simulink model "Casc_Filter_x4"  (Simulink 6.6)
settings: Solver=ode45  StartTime=0.0  StopTime=4100/sampling_freq  RelTol=1e-3
values from neighbouring files (symbols this model uses):
  filter_clk = sampling_freq*clk_mult    (= 144000000)    [Casecade_Taps.m]
  h_g = round(h_g*2^17)/2^17    [Casecade_Taps.m]
  h_k = round(h_k*2^17)/2^17    [Casecade_Taps.m]
  sampling_freq = 48e6    (= 48000000)    [Casecade_Taps.m]
undefined symbols (not defined in the file or in its folder): A, B, Fs, get, PCIN
libraries: xbsIndex_r4 x839, dspsnks4 x5, dspsrcs4 x1, simulink x1
(part 1 of 8)
settings Model: Creator=tbrimeye  LastModifiedBy=tbrimeye
settings DebuggingCC: SignalResolutionControl=TryResolveAllWithWarning  MultiTaskDSMMsg=warning  MultiTaskCondExecSysMsg=none
settings RTWCC: IncludeERTFirstTime=on

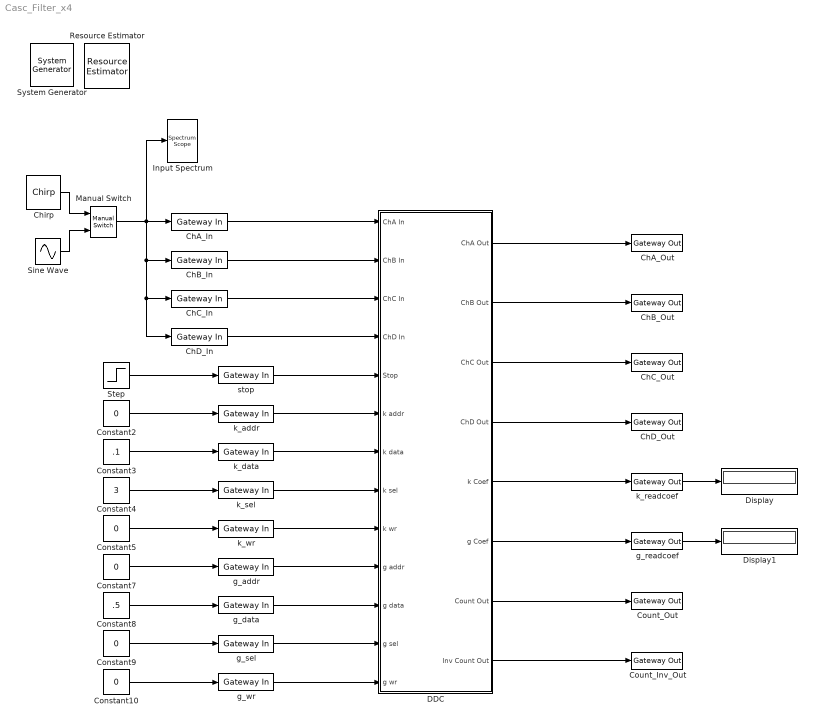
== system Casc_Filter_x4 ==
  " System Generator" : xbsIndex_r4/ System Generator  Tag=genX  SystemSampleTime=-1  xilinxfamily=virtex4  part=xc4vsx35  speed=-11  package=ff668  synthesis_tool=XST  directory=C:/Work_Projects/Xilinx/SysGen_Outputs/DDC_Filters/Casc_Filter_x4_Temp  testbench=off  simulink_period=1/filter_clk  sysclk_period=(1/filter_clk)*1e9  incr_netlist=off  trim_vbits=Everywhere in SubSystem  dbl_ovrd=According to Block Masks  core_generation=According to Block Masks  run_coregen=off  deprecated_control=off  eval_field=0  block_type=sysgen
      settings: block_version=8.2
  ChA_In : xbsIndex_r4/Gateway In  arith_type="Signed  (2's comp)"  n_bits=14  bin_pt=13  quantization="Round  (unbiased: +/- Inf)"  overflow=Saturate  period=1/sampling_freq  dbl_ovrd=off  timing_constraint=None  locs_specified=off  LOCs={}  block_type=gatewayin
      settings: infoedit="Gateway in block.  Converts inputs of type Simulink integer, double and fixed point to  Xilinx fixed point type.<P><P>Hardware notes:  In hardware these blocks become top level input ports."  xl_area=[0 0 0 0 14 0 0]  block_version=8.2
  ChA_Out : xbsIndex_r4/Gateway Out  hdl_port=on  timing_constraint=None  locs_specified=off  LOCs={}  block_type=gatewayout
      settings: infoedit="Gateway out block.  Converts Xilinx fixed point inputs into ouputs of type Simulink integer, double, or fixed point.<P><P>Hardware notes:  In hardware these blocks become top level output ports or are discarded, depending on how they are configured."  xl_area=[0 0 0 0 16 0 0]  block_version=8.2
  ChB_In : xbsIndex_r4/Gateway In  arith_type="Signed  (2's comp)"  n_bits=14  bin_pt=13  quantization="Round  (unbiased: +/- Inf)"  overflow=Saturate  period=1/sampling_freq  dbl_ovrd=off  timing_constraint=None  locs_specified=off  LOCs={}  block_type=gatewayin
      settings: infoedit="Gateway in block.  Converts inputs of type Simulink integer, double and fixed point to  Xilinx fixed point type.<P><P>Hardware notes:  In hardware these blocks become top level input ports."  xl_area=[0 0 0 0 14 0 0]  block_version=8.2
  ChB_Out : xbsIndex_r4/Gateway Out  hdl_port=on  timing_constraint=None  locs_specified=off  LOCs={}  block_type=gatewayout
      settings: infoedit="Gateway out block.  Converts Xilinx fixed point inputs into ouputs of type Simulink integer, double, or fixed point.<P><P>Hardware notes:  In hardware these blocks become top level output ports or are discarded, depending on how they are configured."  xl_area=[0 0 0 0 16 0 0]  block_version=8.2
  ChC_In : xbsIndex_r4/Gateway In  arith_type="Signed  (2's comp)"  n_bits=14  bin_pt=13  quantization="Round  (unbiased: +/- Inf)"  overflow=Saturate  period=1/sampling_freq  dbl_ovrd=off  timing_constraint=None  locs_specified=off  LOCs={}  block_type=gatewayin
      settings: infoedit="Gateway in block.  Converts inputs of type Simulink integer, double and fixed point to  Xilinx fixed point type.<P><P>Hardware notes:  In hardware these blocks become top level input ports."  xl_area=[0 0 0 0 14 0 0]  block_version=8.2
  ChC_Out : xbsIndex_r4/Gateway Out  hdl_port=on  timing_constraint=None  locs_specified=off  LOCs={}  block_type=gatewayout
      settings: infoedit="Gateway out block.  Converts Xilinx fixed point inputs into ouputs of type Simulink integer, double, or fixed point.<P><P>Hardware notes:  In hardware these blocks become top level output ports or are discarded, depending on how they are configured."  xl_area=[0 0 0 0 16 0 0]  block_version=8.2
  ChD_In : xbsIndex_r4/Gateway In  arith_type="Signed  (2's comp)"  n_bits=14  bin_pt=13  quantization="Round  (unbiased: +/- Inf)"  overflow=Saturate  period=1/sampling_freq  dbl_ovrd=off  timing_constraint=None  locs_specified=off  LOCs={}  block_type=gatewayin
      settings: infoedit="Gateway in block.  Converts inputs of type Simulink integer, double and fixed point to  Xilinx fixed point type.<P><P>Hardware notes:  In hardware these blocks become top level input ports."  xl_area=[0 0 0 0 14 0 0]  block_version=8.2
  ChD_Out : xbsIndex_r4/Gateway Out  hdl_port=on  timing_constraint=None  locs_specified=off  LOCs={}  block_type=gatewayout
      settings: infoedit="Gateway out block.  Converts Xilinx fixed point inputs into ouputs of type Simulink integer, double, or fixed point.<P><P>Hardware notes:  In hardware these blocks become top level output ports or are discarded, depending on how they are configured."  xl_area=[0 0 0 0 16 0 0]  block_version=8.2
  Chirp : dspsrcs4/Chirp  sweep=Linear  mode=Unidirectional  f0=0  f1=sampling_freq_div2  t1=4096/sampling_freq  Tsweep=4096/sampling_freq  phase=pi/4  Ts=1/sampling_freq  spf=1  datatype=Double
  Constant{2,5,7,9..10} (5 alike) : Constant  Value=0
  Constant3 : Constant  Value=.1
  Constant4 : Constant  Value=3
  Constant8 : Constant  Value=.5
  Count_Inv_Out : xbsIndex_r4/Gateway Out  hdl_port=on  timing_constraint=None  locs_specified=off  LOCs={}  block_type=gatewayout
      settings: infoedit="Gateway out block.  Converts Xilinx fixed point inputs into ouputs of type Simulink integer, double, or fixed point.<P><P>Hardware notes:  In hardware these blocks become top level output ports or are discarded, depending on how they are configured."  xl_area=[0 0 0 0 16 0 0]  block_version=8.2
  Count_Out : xbsIndex_r4/Gateway Out  hdl_port=on  timing_constraint=None  locs_specified=off  LOCs={}  block_type=gatewayout
      settings: infoedit="Gateway out block.  Converts Xilinx fixed point inputs into ouputs of type Simulink integer, double, or fixed point.<P><P>Hardware notes:  In hardware these blocks become top level output ports or are discarded, depending on how they are configured."  xl_area=[0 0 0 0 16 0 0]  block_version=8.2
  DDC : Subsystem
  Display : Display
  Display1 : Display
  Input Spectrum : dspsnks4/Spectrum Scope  DialogController=dspdialog.SpectrumScope  DialogControllerArgs=DataTag5  SystemSampleTime=-1  ScopeProperties=on  Domain=Frequency  HorizSpan=1  UseBuffer=on  BufferSize=4096  Overlap=64  inpFftLenInherit=on  FFTlength=4096  numAvg=2  DisplayProperties=off  AxisGrid=on  Memory=off  FrameNumber=on  AxisLegend=off  AxisZoom=off  OpenScopeAtSimStart=on  OpenScopeImmediately=off  FigPos=get(0,'defaultfigureposition')  AxisProperties=off  XUnits=Hertz  XRange=[-Fs/2...Fs/2]  InheritXIncr=on  XIncr=1.0  XLabel=Samples  XLimit=Auto  YUnits=dB  XMax=1  XMin=0  YLabel=Magnitude-squared, dB  LineProperties=off  wintypeSpecScope=Boxcar  RsSpecScope=50  betaSpecScope=5  winsampSpecScope=Periodic
      settings: YMin=-100  YMax=0
  Manual Switch : simulink/Signal Routing/Manual Switch  SystemSampleTime=-1  sw=1  action=0  varsize=off
  Resource Estimator : xbsIndex_r4/Resource Estimator  Tag=resEstTag  Slices=925  FFs=1405  BRAMs=7  LUTs=1104  IOBs=133  EBMs=14  TBUFs=0  xl_use_estimator_area=off  est_options=Post Map  xl_estimator_area=[1915 2342 0 3405 33 4 0]  block_type=resource_estimator
      settings: AttributesFormatString=Resource\nEstimator  block_version=8.2
  Sine Wave : Sin  Amplitude=.99  Frequency=2*pi*61e6  SampleTime=1/48e6
  Step : Step  Time=101/filter_clk  Before=1  After=0  SampleTime=1/filter_clk
  g_addr : xbsIndex_r4/Gateway In  arith_type=Unsigned  n_bits=4  bin_pt=0  quantization="Round  (unbiased: +/- Inf)"  overflow=Saturate  period=1/sampling_freq  dbl_ovrd=off  timing_constraint=None  locs_specified=off  LOCs={}  block_type=gatewayin
      settings: infoedit="Gateway in block.  Converts inputs of type Simulink integer, double and fixed point to  Xilinx fixed point type.<P><P>Hardware notes:  In hardware these blocks become top level input ports."  xl_area=[0 0 0 0 4 0 0]  block_version=VER_STRING_GOES_HERE
  g_data : xbsIndex_r4/Gateway In  arith_type="Signed  (2's comp)"  n_bits=18  bin_pt=17  quantization="Round  (unbiased: +/- Inf)"  overflow=Saturate  period=1/sampling_freq  dbl_ovrd=off  timing_constraint=None  locs_specified=off  LOCs={}  block_type=gatewayin
      settings: infoedit="Gateway in block.  Converts inputs of type Simulink integer, double and fixed point to  Xilinx fixed point type.<P><P>Hardware notes:  In hardware these blocks become top level input ports."  xl_area=[0 0 0 0 18 0 0]  block_version=VER_STRING_GOES_HERE
  g_readcoef : xbsIndex_r4/Gateway Out  hdl_port=on  timing_constraint=None  locs_specified=off  LOCs={}  block_type=gatewayout
      settings: infoedit="Gateway out block.  Converts Xilinx fixed point inputs into ouputs of type Simulink integer, double, or fixed point.<P><P>Hardware notes:  In hardware these blocks become top level output ports or are discarded, depending on how they are configured."  xl_area=[0 0 0 0 18 0 0]  block_version=VER_STRING_GOES_HERE
  g_sel : xbsIndex_r4/Gateway In  arith_type=Unsigned  n_bits=2  bin_pt=0  quantization="Round  (unbiased: +/- Inf)"  overflow=Saturate  period=1/sampling_freq  dbl_ovrd=off  timing_constraint=None  locs_specified=off  LOCs={}  block_type=gatewayin
      settings: infoedit="Gateway in block.  Converts inputs of type Simulink integer, double and fixed point to  Xilinx fixed point type.<P><P>Hardware notes:  In hardware these blocks become top level input ports."  xl_area=[0 0 0 0 2 0 0]  block_version=VER_STRING_GOES_HERE
  g_wr : xbsIndex_r4/Gateway In  arith_type=Boolean  n_bits=4  bin_pt=0  quantization="Round  (unbiased: +/- Inf)"  overflow=Saturate  period=1/sampling_freq  dbl_ovrd=off  timing_constraint=None  locs_specified=off  LOCs={}  block_type=gatewayin
      settings: infoedit="Gateway in block.  Converts inputs of type Simulink integer, double and fixed point to  Xilinx fixed point type.<P><P>Hardware notes:  In hardware these blocks become top level input ports."  xl_area=[0 0 0 0 1 0 0]  block_version=VER_STRING_GOES_HERE
  k_addr : xbsIndex_r4/Gateway In  arith_type=Unsigned  n_bits=4  bin_pt=0  quantization="Round  (unbiased: +/- Inf)"  overflow=Saturate  period=1/sampling_freq  dbl_ovrd=off  timing_constraint=None  locs_specified=off  LOCs={}  block_type=gatewayin
      settings: infoedit="Gateway in block.  Converts inputs of type Simulink integer, double and fixed point to  Xilinx fixed point type.<P><P>Hardware notes:  In hardware these blocks become top level input ports."  xl_area=[0 0 0 0 4 0 0]  block_version=VER_STRING_GOES_HERE
  k_data : xbsIndex_r4/Gateway In  arith_type="Signed  (2's comp)"  n_bits=18  bin_pt=17  quantization="Round  (unbiased: +/- Inf)"  overflow=Saturate  period=1/sampling_freq  dbl_ovrd=off  timing_constraint=None  locs_specified=off  LOCs={}  block_type=gatewayin
      settings: infoedit="Gateway in block.  Converts inputs of type Simulink integer, double and fixed point to  Xilinx fixed point type.<P><P>Hardware notes:  In hardware these blocks become top level input ports."  xl_area=[0 0 0 0 18 0 0]  block_version=VER_STRING_GOES_HERE
  k_readcoef : xbsIndex_r4/Gateway Out  hdl_port=on  timing_constraint=None  locs_specified=off  LOCs={}  block_type=gatewayout
      settings: infoedit="Gateway out block.  Converts Xilinx fixed point inputs into ouputs of type Simulink integer, double, or fixed point.<P><P>Hardware notes:  In hardware these blocks become top level output ports or are discarded, depending on how they are configured."  xl_area=[0 0 0 0 18 0 0]  block_version=VER_STRING_GOES_HERE
  k_sel : xbsIndex_r4/Gateway In  arith_type=Unsigned  n_bits=2  bin_pt=0  quantization="Round  (unbiased: +/- Inf)"  overflow=Saturate  period=1/sampling_freq  dbl_ovrd=off  timing_constraint=None  locs_specified=off  LOCs={}  block_type=gatewayin
      settings: infoedit="Gateway in block.  Converts inputs of type Simulink integer, double and fixed point to  Xilinx fixed point type.<P><P>Hardware notes:  In hardware these blocks become top level input ports."  xl_area=[0 0 0 0 2 0 0]  block_version=VER_STRING_GOES_HERE
  k_wr : xbsIndex_r4/Gateway In  arith_type=Boolean  n_bits=4  bin_pt=0  quantization="Round  (unbiased: +/- Inf)"  overflow=Saturate  period=1/sampling_freq  dbl_ovrd=off  timing_constraint=None  locs_specified=off  LOCs={}  block_type=gatewayin
      settings: infoedit="Gateway in block.  Converts inputs of type Simulink integer, double and fixed point to  Xilinx fixed point type.<P><P>Hardware notes:  In hardware these blocks become top level input ports."  xl_area=[0 0 0 0 1 0 0]  block_version=VER_STRING_GOES_HERE
  stop : xbsIndex_r4/Gateway In  arith_type=Unsigned  n_bits=1  bin_pt=0  quantization="Round  (unbiased: +/- Inf)"  overflow=Saturate  period=1/12e6  dbl_ovrd=off  timing_constraint=None  locs_specified=off  LOCs={}  block_type=gatewayin
      settings: infoedit="Gateway in block.  Converts inputs of type Simulink integer, double and fixed point to  Xilinx fixed point type.<P><P>Hardware notes:  In hardware these blocks become top level input ports."  xl_area=[0 0 0 0 1 0 0]  block_version=VER_STRING_GOES_HERE
  wires:
  Chirp/1 -> Manual Switch/1
  Sine Wave/1 -> Manual Switch/2
  ChA_In/1 -> DDC/1(ChA In)
  Manual Switch/1 -> Input Spectrum/1, ChA_In/1, ChB_In/1, ChC_In/1, ChD_In/1
  k_sel/1 -> DDC/8(k sel)
  k_addr/1 -> DDC/6(k addr)
  k_data/1 -> DDC/7(k data)
  k_wr/1 -> DDC/9(k wr)
  DDC/5(k Coef) -> k_readcoef/1
  Constant2/1 -> k_addr/1
  Constant3/1 -> k_data/1
  Constant4/1 -> k_sel/1
  Constant5/1 -> k_wr/1
  k_readcoef/1 -> Display/1
  g_readcoef/1 -> Display1/1
  DDC/6(g Coef) -> g_readcoef/1
  g_addr/1 -> DDC/10(g addr)
  g_data/1 -> DDC/11(g data)
  g_sel/1 -> DDC/12(g sel)
  g_wr/1 -> DDC/13(g wr)
  Constant7/1 -> g_addr/1
  Constant8/1 -> g_data/1
  Constant9/1 -> g_sel/1
  Constant10/1 -> g_wr/1
  DDC/1(ChA Out) -> ChA_Out/1
  stop/1 -> DDC/5(Stop)
  DDC/2(ChB Out) -> ChB_Out/1
  DDC/4(ChD Out) -> ChD_Out/1
  DDC/3(ChC Out) -> ChC_Out/1
  ChB_In/1 -> DDC/2(ChB In)
  ChC_In/1 -> DDC/3(ChC In)
  ChD_In/1 -> DDC/4(ChD In)
  Step/1 -> stop/1
  DDC/7(Count Out) -> Count_Out/1
  DDC/8(Inv Count Out) -> Count_Inv_Out/1

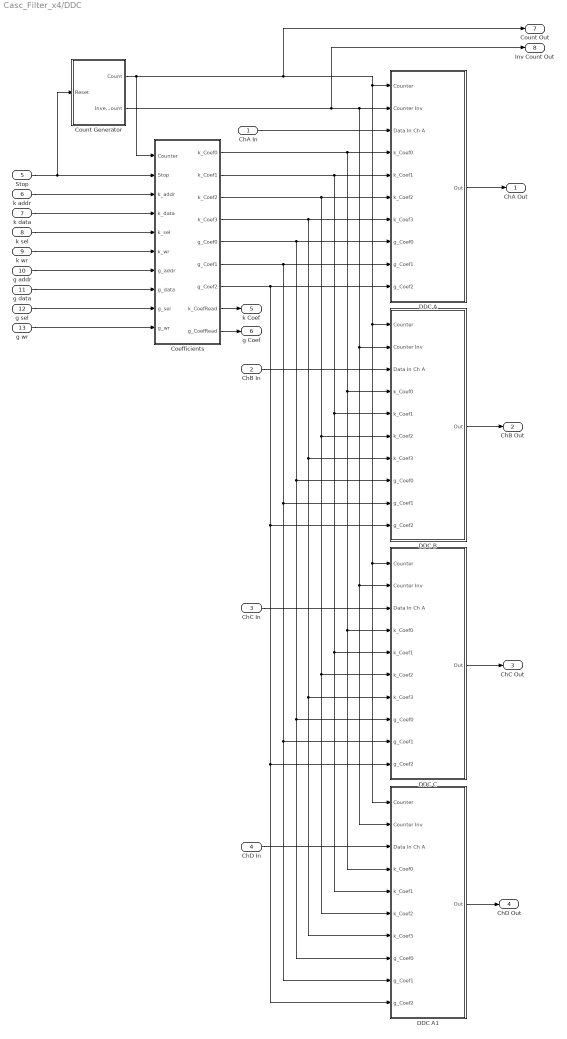
== system Casc_Filter_x4/DDC ==
  ChA In : Inport
  ChB In : Inport  Port=2
  ChC In : Inport  Port=3
  ChD In : Inport  Port=4
  Stop : Inport  Port=5
  k addr : Inport  Port=6
  k data : Inport  Port=7
  k sel : Inport  Port=8
  k wr : Inport  Port=9
  g addr : Inport  Port=10
  g data : Inport  Port=11
  g sel : Inport  Port=12
  g wr : Inport  Port=13
  Coefficients : Subsystem
  Count Generator : Subsystem
  DDC A : Subsystem
  DDC A1 : Subsystem
  DDC B : Subsystem
  DDC C : Subsystem
  ChA Out : Outport
  ChB Out : Outport  Port=2
  ChC Out : Outport  Port=3
  ChD Out : Outport  Port=4
  k Coef : Outport  Port=5
  g Coef : Outport  Port=6
  Count Out : Outport  Port=7
  Inv Count Out : Outport  Port=8
  wires:
  Count Generator/1(Count) -> Coefficients/1(Counter), DDC C/1(Counter), DDC A1/1(Counter), DDC B/1(Counter), DDC A/1(Counter), Count Out/1
  Coefficients/1(k_Coef0) -> DDC C/4(k_Coef0), DDC A1/4(k_Coef0), DDC B/4(k_Coef0), DDC A/4(k_Coef0)
  Coefficients/2(k_Coef1) -> DDC C/5(k_Coef1), DDC A1/5(k_Coef1), DDC B/5(k_Coef1), DDC A/5(k_Coef1)
  Coefficients/3(k_Coef2) -> DDC C/6(k_Coef2), DDC A1/6(k_Coef2), DDC B/6(k_Coef2), DDC A/6(k_Coef2)
  Coefficients/4(k_Coef3) -> DDC C/7(k_Coef3), DDC A1/7(k_Coef3), DDC B/7(k_Coef3), DDC A/7(k_Coef3)
  Count Generator/2(Invert Count) -> DDC C/2(Counter Inv), DDC A1/2(Counter Inv), DDC B/2(Counter Inv), DDC A/2(Counter Inv), Inv Count Out/1
  Coefficients/5(g_Coef0) -> DDC C/8(g_Coef0), DDC A1/8(g_Coef0), DDC B/8(g_Coef0), DDC A/8(g_Coef0)
  Coefficients/6(g_Coef1) -> DDC C/9(g_Coef1), DDC A1/9(g_Coef1), DDC B/9(g_Coef1), DDC A/9(g_Coef1)
  Coefficients/7(g_Coef2) -> DDC C/10(g_Coef2), DDC A1/10(g_Coef2), DDC B/10(g_Coef2), DDC A/10(g_Coef2)
  ChA In/1 -> DDC A/3(Data In Ch A)
  Stop/1 -> Coefficients/2(Stop), Count Generator/1(Reset)
  k addr/1 -> Coefficients/3(k_addr)
  k data/1 -> Coefficients/4(k_data)
  k sel/1 -> Coefficients/5(k_sel)
  k wr/1 -> Coefficients/6(k_wr)
  g addr/1 -> Coefficients/7(g_addr)
  g data/1 -> Coefficients/8(g_data)
  Coefficients/8(k_CoefRead) -> k Coef/1
  g sel/1 -> Coefficients/9(g_sel)
  g wr/1 -> Coefficients/10(g_wr)
  Coefficients/9(g_CoefRead) -> g Coef/1
  DDC A/1(Out) -> ChA Out/1
  DDC B/1(Out) -> ChB Out/1
  DDC C/1(Out) -> ChC Out/1
  DDC A1/1(Out) -> ChD Out/1
  ChB In/1 -> DDC B/3(Data In Ch A)
  ChC In/1 -> DDC C/3(Data In Ch A)
  ChD In/1 -> DDC A1/3(Data In Ch A)

== system Casc_Filter_x4/DDC/Coefficients ==
  Counter : Inport
  Stop : Inport  Port=2
  k_addr : Inport  Port=3
  k_data : Inport  Port=4
  k_sel : Inport  Port=5
  k_wr : Inport  Port=6
  g_addr : Inport  Port=7
  g_data : Inport  Port=8
  g_sel : Inport  Port=9
  g_wr : Inport  Port=10
  Gaus Coef Mem : Subsystem
  Poly Coef Mem : Subsystem
  k_Coef0 : Outport
  k_Coef1 : Outport  Port=2
  k_Coef2 : Outport  Port=3
  k_Coef3 : Outport  Port=4
  g_Coef0 : Outport  Port=5
  g_Coef1 : Outport  Port=6
  g_Coef2 : Outport  Port=7
  k_CoefRead : Outport  Port=8
  g_CoefRead : Outport  Port=9
  wires:
  Stop/1 -> Gaus Coef Mem/1(Stop), Poly Coef Mem/1(Stop)
  Counter/1 -> Poly Coef Mem/2(Counter), Gaus Coef Mem/2(Counter)
  Poly Coef Mem/1(Coef0) -> k_Coef0/1
  Poly Coef Mem/2(Coef1) -> k_Coef1/1
  k_addr/1 -> Poly Coef Mem/3(Addr)
  Poly Coef Mem/3(Coef2) -> k_Coef2/1
  k_data/1 -> Poly Coef Mem/4(Data)
  Poly Coef Mem/4(Coef3) -> k_Coef3/1
  k_sel/1 -> Poly Coef Mem/5(Sel)
  Poly Coef Mem/5(Read) -> k_CoefRead/1
  k_wr/1 -> Poly Coef Mem/6(Wr/R)
  Gaus Coef Mem/1(Coef0) -> g_Coef0/1
  Gaus Coef Mem/2(Coef1) -> g_Coef1/1
  g_addr/1 -> Gaus Coef Mem/3(Addr)
  g_data/1 -> Gaus Coef Mem/4(Data)
  Gaus Coef Mem/3(Coef2) -> g_Coef2/1
  g_sel/1 -> Gaus Coef Mem/5(Sel)
  Gaus Coef Mem/4(Read) -> g_CoefRead/1
  g_wr/1 -> Gaus Coef Mem/6(Wr/R)

== system Casc_Filter_x4/DDC/Count Generator ==
  Reset : Inport
  AddSub : xbsIndex_r4/AddSub  mode=Subtraction  use_carryin=off  use_carryout=off  en=off  latency=0  precision=User Defined  arith_type=Unsigned  n_bits=4  bin_pt=0  quantization=Truncate  overflow=Wrap  dbl_ovrd=off  use_behavioral_HDL=off  pipelined=off  use_rpm=on  block_type=addsub
      settings: block_version=9.2.01
  Constant : xbsIndex_r4/Constant  arith_type=Unsigned  const=11  n_bits=4  bin_pt=0  explicit_period=off  period=1  equ=P=C  opselect=C  inp2=PCIN>>17  opr=+  inp1=P  carry=CIN  dbl_ovrd=off  block_type=constant
      settings: block_version=9.2.01
  Convert : xbsIndex_r4/Convert  arith_type=Boolean  n_bits=16  bin_pt=14  quantization=Truncate  overflow=Wrap  latency=0  dbl_ovrd=off  pipeline=off  block_type=convert
      settings: block_version=9.2.01
  Counter : xbsIndex_r4/Counter  cnt_type=Count Limited  cnt_to=11  operation=Up  start_count=0  cnt_by_val=1  arith_type=Unsigned  n_bits=4  bin_pt=0  load_pin=off  rst=on  en=off  explicit_period=on  period=1/filter_clk  dbl_ovrd=off  use_behavioral_HDL=off  use_rpm=off  block_type=counter
      settings: block_version=8.2
  Count : Outport
  Invert Count : Outport  Port=2
  wires:
  Counter/1 -> AddSub/2, Count/1
  Constant/1 -> AddSub/1
  Convert/1 -> Counter/1
  Reset/1 -> Convert/1
  AddSub/1 -> Invert Count/1

== system Casc_Filter_x4/DDC/DDC A ==
  Counter : Inport
  Counter Inv : Inport  Port=2
  Data In Ch A : Inport  Port=3
  k_Coef0 : Inport  Port=4
  k_Coef1 : Inport  Port=5
  k_Coef2 : Inport  Port=6
  k_Coef3 : Inport  Port=7
  g_Coef0 : Inport  Port=8
  g_Coef1 : Inport  Port=9
  g_Coef2 : Inport  Port=10
  Concat : xbsIndex_r4/Concat  num_inputs=2  dbl_ovrd=off  block_type=concat
      settings: block_version=8.2
  Gateway Out : xbsIndex_r4/Gateway Out  hdl_port=off  timing_constraint=None  locs_specified=off  LOCs={}  block_type=gatewayout
      settings: infoedit="Gateway out block.  Converts Xilinx fixed point inputs into ouputs of type Simulink integer, double, or fixed point.<P><P>Hardware notes:  In hardware these blocks become top level output ports or are discarded, depending on how they are configured."  block_version=8.2
  Gateway Out1 : xbsIndex_r4/Gateway Out  hdl_port=off  timing_constraint=None  locs_specified=off  LOCs={}  block_type=gatewayout
      settings: infoedit="Gateway out block.  Converts Xilinx fixed point inputs into ouputs of type Simulink integer, double, or fixed point.<P><P>Hardware notes:  In hardware these blocks become top level output ports or are discarded, depending on how they are configured."  block_version=8.2
  Gaussian FIR Filters : Subsystem
  Poly Spectrum : dspsnks4/Spectrum Scope  DialogController=dspdialog.SpectrumScope  DialogControllerArgs=DataTag1  SystemSampleTime=-1  ScopeProperties=on  Domain=Frequency  HorizSpan=1  UseBuffer=on  BufferSize=1024  Overlap=64  inpFftLenInherit=on  FFTlength=1024  numAvg=2  DisplayProperties=off  AxisGrid=on  Memory=off  FrameNumber=on  AxisLegend=off  AxisZoom=off  OpenScopeAtSimStart=on  OpenScopeImmediately=off  FigPos=get(0,'defaultfigureposition')  AxisProperties=off  XUnits=Hertz  XRange=[-Fs/2...Fs/2]  InheritXIncr=on  XIncr=1.0  XLabel=Samples  XLimit=Auto  YUnits=dB  XMax=1  XMin=0  YLabel=Magnitude-squared, dB  LineProperties=off  wintypeSpecScope=Boxcar  RsSpecScope=50  betaSpecScope=5  winsampSpecScope=Periodic
      settings: YMin=-120  YMax=0
  Polyphase Kaiser FIR Filter : Subsystem
  Real-Imag to Complex1 : RealImagToComplex
  Reinterpret : xbsIndex_r4/Reinterpret  force_arith_type=on  arith_type=Unsigned  force_bin_pt=on  bin_pt=0  block_type=reinterpret
      settings: infoedit="Changes signal type without altering the binary representation.   You can changed the signal between signed and unsigned, and relocate the binary point.<P><P>Hardware notes: In hardware this block costs nothing.<P><P>Example:  Suppose the input is 6 bits wide, signed, with 2 fractional bits, and the output is forced to unsigned with 0 fractional bits.  Then an input of -2.0 (1110.00 in binary 2's complement) becomes an output of 56 (111000 in binary)."  block_version=8.2
  Reinterpret1 : xbsIndex_r4/Reinterpret  force_arith_type=on  arith_type=Unsigned  force_bin_pt=on  bin_pt=0  block_type=reinterpret
      settings: infoedit="Changes signal type without altering the binary representation.   You can changed the signal between signed and unsigned, and relocate the binary point.<P><P>Hardware notes: In hardware this block costs nothing.<P><P>Example:  Suppose the input is 6 bits wide, signed, with 2 fractional bits, and the output is forced to unsigned with 0 fractional bits.  Then an input of -2.0 (1110.00 in binary 2's complement) becomes an output of 56 (111000 in binary)."  block_version=8.2
  Scope1 : Scope  NumInputPorts=2
      settings: YMin=-5~-5  YMax=5~5  SaveName=ScopeData3
  Out : Outport
  wires:
  Counter Inv/1 -> Polyphase Kaiser FIR Filter/2(Counter Inv), Gaussian FIR Filters/2(Counter Inv)
  Real-Imag to Complex1/1 -> Poly Spectrum/1
  Counter/1 -> Polyphase Kaiser FIR Filter/1(Counter), Gaussian FIR Filters/1(Counter)
  Data In Ch A/1 -> Polyphase Kaiser FIR Filter/3(Data In)
  k_Coef0/1 -> Polyphase Kaiser FIR Filter/4(Coef0)
  k_Coef1/1 -> Polyphase Kaiser FIR Filter/5(Coef1)
  k_Coef2/1 -> Polyphase Kaiser FIR Filter/6(Coef2)
  k_Coef3/1 -> Polyphase Kaiser FIR Filter/7(Coef3)
  Polyphase Kaiser FIR Filter/1(Q Out) -> Gaussian FIR Filters/3(Q In), Gateway Out1/1
  Polyphase Kaiser FIR Filter/2(I Out) -> Gaussian FIR Filters/7(I In), Gateway Out/1
  g_Coef0/1 -> Gaussian FIR Filters/4(Coef0)
  g_Coef1/1 -> Gaussian FIR Filters/5(Coef1)
  g_Coef2/1 -> Gaussian FIR Filters/6(Coef2)
  Gateway Out/1 -> Real-Imag to Complex1/1, Scope1/1
  Gateway Out1/1 -> Real-Imag to Complex1/2, Scope1/2
  Reinterpret/1 -> Concat/1
  Reinterpret1/1 -> Concat/2
  Concat/1 -> Out/1
  Gaussian FIR Filters/1(I Out) -> Reinterpret/1
  Gaussian FIR Filters/2(Q Out) -> Reinterpret1/1

== system Casc_Filter_x4/DDC/DDC A1 ==
  Counter : Inport
  Counter Inv : Inport  Port=2
  Data In Ch A : Inport  Port=3
  k_Coef0 : Inport  Port=4
  k_Coef1 : Inport  Port=5
  k_Coef2 : Inport  Port=6
  k_Coef3 : Inport  Port=7
  g_Coef0 : Inport  Port=8
  g_Coef1 : Inport  Port=9
  g_Coef2 : Inport  Port=10
  Concat : xbsIndex_r4/Concat  num_inputs=2  dbl_ovrd=off  block_type=concat
      settings: block_version=8.2
  Gateway Out : xbsIndex_r4/Gateway Out  hdl_port=off  timing_constraint=None  locs_specified=off  LOCs={}  block_type=gatewayout
      settings: infoedit="Gateway out block.  Converts Xilinx fixed point inputs into ouputs of type Simulink integer, double, or fixed point.<P><P>Hardware notes:  In hardware these blocks become top level output ports or are discarded, depending on how they are configured."  block_version=8.2
  Gateway Out1 : xbsIndex_r4/Gateway Out  hdl_port=off  timing_constraint=None  locs_specified=off  LOCs={}  block_type=gatewayout
      settings: infoedit="Gateway out block.  Converts Xilinx fixed point inputs into ouputs of type Simulink integer, double, or fixed point.<P><P>Hardware notes:  In hardware these blocks become top level output ports or are discarded, depending on how they are configured."  block_version=8.2
  Gaussian FIR Filters : Subsystem
  Poly Spectrum : dspsnks4/Spectrum Scope  DialogController=dspdialog.SpectrumScope  DialogControllerArgs=DataTag2  SystemSampleTime=-1  ScopeProperties=on  Domain=Frequency  HorizSpan=1  UseBuffer=on  BufferSize=1024  Overlap=64  inpFftLenInherit=on  FFTlength=1024  numAvg=2  DisplayProperties=off  AxisGrid=on  Memory=off  FrameNumber=on  AxisLegend=off  AxisZoom=off  OpenScopeAtSimStart=on  OpenScopeImmediately=off  FigPos=get(0,'defaultfigureposition')  AxisProperties=off  XUnits=Hertz  XRange=[-Fs/2...Fs/2]  InheritXIncr=on  XIncr=1.0  XLabel=Samples  XLimit=Auto  YUnits=dB  XMax=1  XMin=0  YLabel=Magnitude-squared, dB  LineProperties=off  wintypeSpecScope=Boxcar  RsSpecScope=50  betaSpecScope=5  winsampSpecScope=Periodic
      settings: YMin=-120  YMax=0
  Polyphase Kaiser FIR Filter : Subsystem
  Real-Imag to Complex1 : RealImagToComplex
  Reinterpret : xbsIndex_r4/Reinterpret  force_arith_type=on  arith_type=Unsigned  force_bin_pt=on  bin_pt=0  block_type=reinterpret
      settings: infoedit="Changes signal type without altering the binary representation.   You can changed the signal between signed and unsigned, and relocate the binary point.<P><P>Hardware notes: In hardware this block costs nothing.<P><P>Example:  Suppose the input is 6 bits wide, signed, with 2 fractional bits, and the output is forced to unsigned with 0 fractional bits.  Then an input of -2.0 (1110.00 in binary 2's complement) becomes an output of 56 (111000 in binary)."  block_version=8.2
  Reinterpret1 : xbsIndex_r4/Reinterpret  force_arith_type=on  arith_type=Unsigned  force_bin_pt=on  bin_pt=0  block_type=reinterpret
      settings: infoedit="Changes signal type without altering the binary representation.   You can changed the signal between signed and unsigned, and relocate the binary point.<P><P>Hardware notes: In hardware this block costs nothing.<P><P>Example:  Suppose the input is 6 bits wide, signed, with 2 fractional bits, and the output is forced to unsigned with 0 fractional bits.  Then an input of -2.0 (1110.00 in binary 2's complement) becomes an output of 56 (111000 in binary)."  block_version=8.2
  Scope1 : Scope  NumInputPorts=2
      settings: YMin=-5~-5  YMax=5~5  SaveName=ScopeData3
  Out : Outport
  wires:
  Counter Inv/1 -> Polyphase Kaiser FIR Filter/2(Counter Inv), Gaussian FIR Filters/2(Counter Inv)
  Real-Imag to Complex1/1 -> Poly Spectrum/1
  Counter/1 -> Polyphase Kaiser FIR Filter/1(Counter), Gaussian FIR Filters/1(Counter)
  Data In Ch A/1 -> Polyphase Kaiser FIR Filter/3(Data In)
  k_Coef0/1 -> Polyphase Kaiser FIR Filter/4(Coef0)
  k_Coef1/1 -> Polyphase Kaiser FIR Filter/5(Coef1)
  k_Coef2/1 -> Polyphase Kaiser FIR Filter/6(Coef2)
  k_Coef3/1 -> Polyphase Kaiser FIR Filter/7(Coef3)
  Polyphase Kaiser FIR Filter/1(Q Out) -> Gaussian FIR Filters/3(Q In), Gateway Out1/1
  Polyphase Kaiser FIR Filter/2(I Out) -> Gaussian FIR Filters/7(I In), Gateway Out/1
  g_Coef0/1 -> Gaussian FIR Filters/4(Coef0)
  g_Coef1/1 -> Gaussian FIR Filters/5(Coef1)
  g_Coef2/1 -> Gaussian FIR Filters/6(Coef2)
  Gateway Out/1 -> Real-Imag to Complex1/1, Scope1/1
  Gateway Out1/1 -> Real-Imag to Complex1/2, Scope1/2
  Reinterpret/1 -> Concat/1
  Reinterpret1/1 -> Concat/2
  Concat/1 -> Out/1
  Gaussian FIR Filters/1(I Out) -> Reinterpret/1
  Gaussian FIR Filters/2(Q Out) -> Reinterpret1/1

== system Casc_Filter_x4/DDC/DDC B ==
  Counter : Inport
  Counter Inv : Inport  Port=2
  Data In Ch A : Inport  Port=3
  k_Coef0 : Inport  Port=4
  k_Coef1 : Inport  Port=5
  k_Coef2 : Inport  Port=6
  k_Coef3 : Inport  Port=7
  g_Coef0 : Inport  Port=8
  g_Coef1 : Inport  Port=9
  g_Coef2 : Inport  Port=10
  Concat : xbsIndex_r4/Concat  num_inputs=2  dbl_ovrd=off  block_type=concat
      settings: block_version=8.2
  Gateway Out : xbsIndex_r4/Gateway Out  hdl_port=off  timing_constraint=None  locs_specified=off  LOCs={}  block_type=gatewayout
      settings: infoedit="Gateway out block.  Converts Xilinx fixed point inputs into ouputs of type Simulink integer, double, or fixed point.<P><P>Hardware notes:  In hardware these blocks become top level output ports or are discarded, depending on how they are configured."  block_version=8.2
  Gateway Out1 : xbsIndex_r4/Gateway Out  hdl_port=off  timing_constraint=None  locs_specified=off  LOCs={}  block_type=gatewayout
      settings: infoedit="Gateway out block.  Converts Xilinx fixed point inputs into ouputs of type Simulink integer, double, or fixed point.<P><P>Hardware notes:  In hardware these blocks become top level output ports or are discarded, depending on how they are configured."  block_version=8.2
  Gaussian FIR Filters : Subsystem
  Poly Spectrum : dspsnks4/Spectrum Scope  DialogController=dspdialog.SpectrumScope  DialogControllerArgs=DataTag3  SystemSampleTime=-1  ScopeProperties=on  Domain=Frequency  HorizSpan=1  UseBuffer=on  BufferSize=1024  Overlap=64  inpFftLenInherit=on  FFTlength=1024  numAvg=2  DisplayProperties=off  AxisGrid=on  Memory=off  FrameNumber=on  AxisLegend=off  AxisZoom=off  OpenScopeAtSimStart=on  OpenScopeImmediately=off  FigPos=get(0,'defaultfigureposition')  AxisProperties=off  XUnits=Hertz  XRange=[-Fs/2...Fs/2]  InheritXIncr=on  XIncr=1.0  XLabel=Samples  XLimit=Auto  YUnits=dB  XMax=1  XMin=0  YLabel=Magnitude-squared, dB  LineProperties=off  wintypeSpecScope=Boxcar  RsSpecScope=50  betaSpecScope=5  winsampSpecScope=Periodic
      settings: YMin=-120  YMax=0
  Polyphase Kaiser FIR Filter : Subsystem
  Real-Imag to Complex1 : RealImagToComplex
  Reinterpret : xbsIndex_r4/Reinterpret  force_arith_type=on  arith_type=Unsigned  force_bin_pt=on  bin_pt=0  block_type=reinterpret
      settings: infoedit="Changes signal type without altering the binary representation.   You can changed the signal between signed and unsigned, and relocate the binary point.<P><P>Hardware notes: In hardware this block costs nothing.<P><P>Example:  Suppose the input is 6 bits wide, signed, with 2 fractional bits, and the output is forced to unsigned with 0 fractional bits.  Then an input of -2.0 (1110.00 in binary 2's complement) becomes an output of 56 (111000 in binary)."  block_version=8.2
  Reinterpret1 : xbsIndex_r4/Reinterpret  force_arith_type=on  arith_type=Unsigned  force_bin_pt=on  bin_pt=0  block_type=reinterpret
      settings: infoedit="Changes signal type without altering the binary representation.   You can changed the signal between signed and unsigned, and relocate the binary point.<P><P>Hardware notes: In hardware this block costs nothing.<P><P>Example:  Suppose the input is 6 bits wide, signed, with 2 fractional bits, and the output is forced to unsigned with 0 fractional bits.  Then an input of -2.0 (1110.00 in binary 2's complement) becomes an output of 56 (111000 in binary)."  block_version=8.2
  Scope1 : Scope  NumInputPorts=2
      settings: YMin=-5~-5  YMax=5~5  SaveName=ScopeData3
  Out : Outport
  wires:
  Counter Inv/1 -> Polyphase Kaiser FIR Filter/2(Counter Inv), Gaussian FIR Filters/2(Counter Inv)
  Real-Imag to Complex1/1 -> Poly Spectrum/1
  Counter/1 -> Polyphase Kaiser FIR Filter/1(Counter), Gaussian FIR Filters/1(Counter)
  Data In Ch A/1 -> Polyphase Kaiser FIR Filter/3(Data In)
  k_Coef0/1 -> Polyphase Kaiser FIR Filter/4(Coef0)
  k_Coef1/1 -> Polyphase Kaiser FIR Filter/5(Coef1)
  k_Coef2/1 -> Polyphase Kaiser FIR Filter/6(Coef2)
  k_Coef3/1 -> Polyphase Kaiser FIR Filter/7(Coef3)
  Polyphase Kaiser FIR Filter/1(Q Out) -> Gaussian FIR Filters/3(Q In), Gateway Out1/1
  Polyphase Kaiser FIR Filter/2(I Out) -> Gaussian FIR Filters/7(I In), Gateway Out/1
  g_Coef0/1 -> Gaussian FIR Filters/4(Coef0)
  g_Coef1/1 -> Gaussian FIR Filters/5(Coef1)
  g_Coef2/1 -> Gaussian FIR Filters/6(Coef2)
  Gateway Out/1 -> Real-Imag to Complex1/1, Scope1/1
  Gateway Out1/1 -> Real-Imag to Complex1/2, Scope1/2
  Reinterpret/1 -> Concat/1
  Reinterpret1/1 -> Concat/2
  Concat/1 -> Out/1
  Gaussian FIR Filters/1(I Out) -> Reinterpret/1
  Gaussian FIR Filters/2(Q Out) -> Reinterpret1/1

== system Casc_Filter_x4/DDC/DDC C ==
  Counter : Inport
  Counter Inv : Inport  Port=2
  Data In Ch A : Inport  Port=3
  k_Coef0 : Inport  Port=4
  k_Coef1 : Inport  Port=5
  k_Coef2 : Inport  Port=6
  k_Coef3 : Inport  Port=7
  g_Coef0 : Inport  Port=8
  g_Coef1 : Inport  Port=9
  g_Coef2 : Inport  Port=10
  Concat : xbsIndex_r4/Concat  num_inputs=2  dbl_ovrd=off  block_type=concat
      settings: block_version=8.2
  Gateway Out : xbsIndex_r4/Gateway Out  hdl_port=off  timing_constraint=None  locs_specified=off  LOCs={}  block_type=gatewayout
      settings: infoedit="Gateway out block.  Converts Xilinx fixed point inputs into ouputs of type Simulink integer, double, or fixed point.<P><P>Hardware notes:  In hardware these blocks become top level output ports or are discarded, depending on how they are configured."  block_version=8.2
  Gateway Out1 : xbsIndex_r4/Gateway Out  hdl_port=off  timing_constraint=None  locs_specified=off  LOCs={}  block_type=gatewayout
      settings: infoedit="Gateway out block.  Converts Xilinx fixed point inputs into ouputs of type Simulink integer, double, or fixed point.<P><P>Hardware notes:  In hardware these blocks become top level output ports or are discarded, depending on how they are configured."  block_version=8.2
  Gaussian FIR Filters : Subsystem
  Poly Spectrum : dspsnks4/Spectrum Scope  DialogController=dspdialog.SpectrumScope  DialogControllerArgs=DataTag4  SystemSampleTime=-1  ScopeProperties=on  Domain=Frequency  HorizSpan=1  UseBuffer=on  BufferSize=1024  Overlap=64  inpFftLenInherit=on  FFTlength=1024  numAvg=2  DisplayProperties=off  AxisGrid=on  Memory=off  FrameNumber=on  AxisLegend=off  AxisZoom=off  OpenScopeAtSimStart=on  OpenScopeImmediately=off  FigPos=get(0,'defaultfigureposition')  AxisProperties=off  XUnits=Hertz  XRange=[-Fs/2...Fs/2]  InheritXIncr=on  XIncr=1.0  XLabel=Samples  XLimit=Auto  YUnits=dB  XMax=1  XMin=0  YLabel=Magnitude-squared, dB  LineProperties=off  wintypeSpecScope=Boxcar  RsSpecScope=50  betaSpecScope=5  winsampSpecScope=Periodic
      settings: YMin=-120  YMax=0
  Polyphase Kaiser FIR Filter : Subsystem
  Real-Imag to Complex1 : RealImagToComplex
  Reinterpret : xbsIndex_r4/Reinterpret  force_arith_type=on  arith_type=Unsigned  force_bin_pt=on  bin_pt=0  block_type=reinterpret
      settings: infoedit="Changes signal type without altering the binary representation.   You can changed the signal between signed and unsigned, and relocate the binary point.<P><P>Hardware notes: In hardware this block costs nothing.<P><P>Example:  Suppose the input is 6 bits wide, signed, with 2 fractional bits, and the output is forced to unsigned with 0 fractional bits.  Then an input of -2.0 (1110.00 in binary 2's complement) becomes an output of 56 (111000 in binary)."  block_version=8.2
  Reinterpret1 : xbsIndex_r4/Reinterpret  force_arith_type=on  arith_type=Unsigned  force_bin_pt=on  bin_pt=0  block_type=reinterpret
      settings: infoedit="Changes signal type without altering the binary representation.   You can changed the signal between signed and unsigned, and relocate the binary point.<P><P>Hardware notes: In hardware this block costs nothing.<P><P>Example:  Suppose the input is 6 bits wide, signed, with 2 fractional bits, and the output is forced to unsigned with 0 fractional bits.  Then an input of -2.0 (1110.00 in binary 2's complement) becomes an output of 56 (111000 in binary)."  block_version=8.2
  Scope1 : Scope  NumInputPorts=2
      settings: YMin=-5~-5  YMax=5~5  SaveName=ScopeData3
  Out : Outport
  wires:
  Counter Inv/1 -> Polyphase Kaiser FIR Filter/2(Counter Inv), Gaussian FIR Filters/2(Counter Inv)
  Real-Imag to Complex1/1 -> Poly Spectrum/1
  Counter/1 -> Polyphase Kaiser FIR Filter/1(Counter), Gaussian FIR Filters/1(Counter)
  Data In Ch A/1 -> Polyphase Kaiser FIR Filter/3(Data In)
  k_Coef0/1 -> Polyphase Kaiser FIR Filter/4(Coef0)
  k_Coef1/1 -> Polyphase Kaiser FIR Filter/5(Coef1)
  k_Coef2/1 -> Polyphase Kaiser FIR Filter/6(Coef2)
  k_Coef3/1 -> Polyphase Kaiser FIR Filter/7(Coef3)
  Polyphase Kaiser FIR Filter/1(Q Out) -> Gaussian FIR Filters/3(Q In), Gateway Out1/1
  Polyphase Kaiser FIR Filter/2(I Out) -> Gaussian FIR Filters/7(I In), Gateway Out/1
  g_Coef0/1 -> Gaussian FIR Filters/4(Coef0)
  g_Coef1/1 -> Gaussian FIR Filters/5(Coef1)
  g_Coef2/1 -> Gaussian FIR Filters/6(Coef2)
  Gateway Out/1 -> Real-Imag to Complex1/1, Scope1/1
  Gateway Out1/1 -> Real-Imag to Complex1/2, Scope1/2
  Reinterpret/1 -> Concat/1
  Reinterpret1/1 -> Concat/2
  Concat/1 -> Out/1
  Gaussian FIR Filters/1(I Out) -> Reinterpret/1
  Gaussian FIR Filters/2(Q Out) -> Reinterpret1/1

== system Casc_Filter_x4/DDC/Coefficients/Gaus Coef Mem ==
  Stop : Inport
  Counter : Inport  Port=2
  Addr : Inport  Port=3
  Data : Inport  Port=4
  Sel : Inport  Port=5
  Wr/R : Inport  Port=6
  Mux : xbsIndex_r4/Mux  inputs=2  en=off  latency=1  precision=Full  arith_type=Unsigned  n_bits=16  bin_pt=14  quantization=Truncate  overflow=Wrap  dbl_ovrd=off  block_type=mux
      settings: xl_area=[2 0 0 4 0 0 0]  block_version=VER_STRING_GOES_HERE
  Mux1 : xbsIndex_r4/Mux  inputs=3  en=on  latency=1  precision=Full  arith_type=Unsigned  n_bits=16  bin_pt=14  quantization=Truncate  overflow=Wrap  dbl_ovrd=off  block_type=mux
      settings: xl_area=[18 18 0 36 0 0 0]  block_version=VER_STRING_GOES_HERE
  Select Decoder : Subsystem
  Single Port RAM : xbsIndex_r4/Single Port RAM  depth=16  initVector=[h_g(1:12),0,0,0,0]  distributed_mem=Block RAM  write_mode=No Read On Write  rst=off  init_reg=0  en=off  latency=11  dbl_ovrd=off  optimize=Area  use_rpm=off  block_type=spram
      settings: xl_area=[18 0 0 36 0 0 0]  block_version=8.2
  Single Port RAM1 : xbsIndex_r4/Single Port RAM  depth=16  initVector=[h_g(13:24),0,0,0,0]  distributed_mem=Block RAM  write_mode=No Read On Write  rst=off  init_reg=0  en=off  latency=11  dbl_ovrd=off  optimize=Area  use_rpm=off  block_type=spram
      settings: xl_area=[18 0 0 36 0 0 0]  block_version=8.2
  Single Port RAM2 : xbsIndex_r4/Single Port RAM  depth=16  initVector=[h_g(25:36),0,0,0,0]  distributed_mem=Block RAM  write_mode=No Read On Write  rst=off  init_reg=0  en=off  latency=11  dbl_ovrd=off  optimize=Area  use_rpm=off  block_type=spram
      settings: xl_area=[18 0 0 36 0 0 0]  block_version=8.2
  Coef0 : Outport
  Coef1 : Outport  Port=2
  Coef2 : Outport  Port=3
  Read : Outport  Port=4
  wires:
  Data/1 -> Single Port RAM1/2, Single Port RAM2/2, Single Port RAM/2
  Single Port RAM/1 -> Mux1/2, Coef0/1
  Single Port RAM1/1 -> Mux1/3, Coef1/1
  Single Port RAM2/1 -> Mux1/4, Coef2/1
  Stop/1 -> Mux/1, Select Decoder/1(Run/Stop)
  Mux/1 -> Single Port RAM/1, Single Port RAM1/1, Single Port RAM2/1
  Mux1/1 -> Read/1
  Counter/1 -> Mux/2
  Addr/1 -> Mux/3
  Sel/1 -> Select Decoder/3(Sel), Mux1/1
  Select Decoder/2(Wr0) -> Single Port RAM/3
  Select Decoder/3(Wr1) -> Single Port RAM1/3
  Select Decoder/4(Wr2) -> Single Port RAM2/3
  Wr/R/1 -> Select Decoder/2(Wr/R)
  Select Decoder/1(R_En) -> Mux1/5

== system Casc_Filter_x4/DDC/Coefficients/Poly Coef Mem ==
  Stop : Inport
  Counter : Inport  Port=2
  Addr : Inport  Port=3
  Data : Inport  Port=4
  Sel : Inport  Port=5
  Wr/R : Inport  Port=6
  Mux : xbsIndex_r4/Mux  inputs=2  en=off  latency=1  precision=Full  arith_type=Unsigned  n_bits=16  bin_pt=14  quantization=Truncate  overflow=Wrap  dbl_ovrd=off  block_type=mux
      settings: xl_area=[2 0 0 4 0 0 0]  block_version=VER_STRING_GOES_HERE
  Mux1 : xbsIndex_r4/Mux  inputs=4  en=on  latency=1  precision=Full  arith_type=Unsigned  n_bits=16  bin_pt=14  quantization=Truncate  overflow=Wrap  dbl_ovrd=off  block_type=mux
      settings: xl_area=[18 18 0 36 0 0 0]  block_version=VER_STRING_GOES_HERE
  Select Decoder : Subsystem
  Single Port RAM : xbsIndex_r4/Single Port RAM  depth=16  initVector=[h_k(1:4:48),0,0,0,0]  distributed_mem=Block RAM  write_mode=No Read On Write  rst=off  init_reg=0  en=off  latency=11  dbl_ovrd=off  optimize=Area  use_rpm=off  block_type=spram
      settings: xl_area=[18 0 0 36 0 0 0]  block_version=8.2
  Single Port RAM1 : xbsIndex_r4/Single Port RAM  depth=16  initVector=[h_k(2:4:48),0,0,0,0]  distributed_mem=Block RAM  write_mode=No Read On Write  rst=off  init_reg=0  en=off  latency=11  dbl_ovrd=off  optimize=Area  use_rpm=off  block_type=spram
      settings: xl_area=[18 0 0 36 0 0 0]  block_version=8.2
  Single Port RAM2 : xbsIndex_r4/Single Port RAM  depth=16  initVector=[h_k(3:4:48),0,0,0,0]  distributed_mem=Block RAM  write_mode=No Read On Write  rst=off  init_reg=0  en=off  latency=11  dbl_ovrd=off  optimize=Area  use_rpm=off  block_type=spram
      settings: xl_area=[18 0 0 36 0 0 0]  block_version=8.2
  Single Port RAM3 : xbsIndex_r4/Single Port RAM  depth=16  initVector=[h_k(4:4:48),0,0,0,0]  distributed_mem=Block RAM  write_mode=No Read On Write  rst=off  init_reg=0  en=off  latency=11  dbl_ovrd=off  optimize=Area  use_rpm=off  block_type=spram
      settings: xl_area=[18 0 0 36 0 0 0]  block_version=8.2
  Coef0 : Outport
  Coef1 : Outport  Port=2
  Coef2 : Outport  Port=3
  Coef3 : Outport  Port=4
  Read : Outport  Port=5
  wires:
  Data/1 -> Single Port RAM2/2, Single Port RAM3/2, Single Port RAM1/2, Single Port RAM/2
  Single Port RAM/1 -> Mux1/2, Coef0/1
  Single Port RAM1/1 -> Mux1/3, Coef1/1
  Single Port RAM2/1 -> Mux1/4, Coef2/1
  Single Port RAM3/1 -> Mux1/5, Coef3/1
  Stop/1 -> Mux/1, Select Decoder/1(Run/Stop)
  Mux/1 -> Single Port RAM1/1, Single Port RAM2/1, Single Port RAM3/1, Single Port RAM/1
  Mux1/1 -> Read/1
  Counter/1 -> Mux/2
  Addr/1 -> Mux/3
  Sel/1 -> Select Decoder/3(Sel), Mux1/1
  Wr/R/1 -> Select Decoder/2(Wr/R)
  Select Decoder/2(Wr0) -> Single Port RAM/3
  Select Decoder/3(Wr1) -> Single Port RAM1/3
  Select Decoder/4(Wr2) -> Single Port RAM2/3
  Select Decoder/5(Wr3) -> Single Port RAM3/3
  Select Decoder/1(R_En) -> Mux1/6

== system Casc_Filter_x4/DDC/DDC A/Gaussian FIR Filters ==
  Counter : Inport
  Counter Inv : Inport  Port=2
  Q In : Inport  Port=3
  Coef0 : Inport  Port=4
  Coef1 : Inport  Port=5
  Coef2 : Inport  Port=6
  I In : Inport  Port=7
  Gaussian FIR Filter : Subsystem
  Gaussian FIR Filter1 : Subsystem
  I Out : Outport
  Q Out : Outport  Port=2
  wires:
  Counter/1 -> Gaussian FIR Filter/1(Counter), Gaussian FIR Filter1/1(Counter)
  Counter Inv/1 -> Gaussian FIR Filter/2(Counter Inv), Gaussian FIR Filter1/2(Counter Inv)
  Q In/1 -> Gaussian FIR Filter/3(Data In)
  I In/1 -> Gaussian FIR Filter1/3(Data In)
  Gaussian FIR Filter/1(Data Out) -> Q Out/1
  Gaussian FIR Filter1/1(Data Out) -> I Out/1
  Coef0/1 -> Gaussian FIR Filter/4(Coef0), Gaussian FIR Filter1/4(Coef0)
  Coef1/1 -> Gaussian FIR Filter/5(Coef1), Gaussian FIR Filter1/5(Coef1)
  Coef2/1 -> Gaussian FIR Filter/6(Coef2), Gaussian FIR Filter1/6(Coef2)

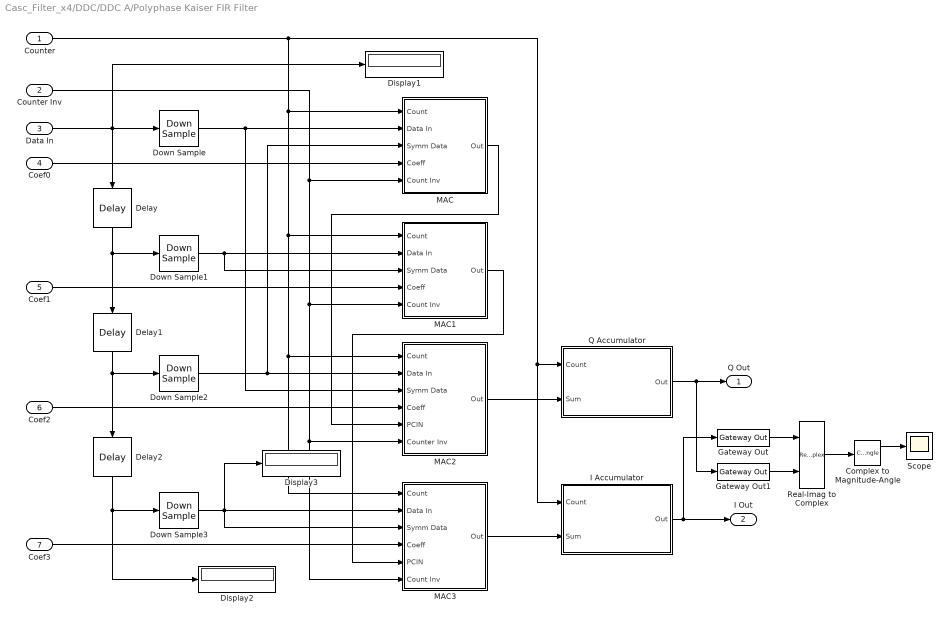
== system Casc_Filter_x4/DDC/DDC A/Polyphase Kaiser FIR Filter ==
  Counter : Inport
  Counter Inv : Inport  Port=2
  Data In : Inport  Port=3
  Coef0 : Inport  Port=4
  Coef1 : Inport  Port=5
  Coef2 : Inport  Port=6
  Coef3 : Inport  Port=7
  Complex to Magnitude-Angle : ComplexToMagnitudeAngle
  Delay : xbsIndex_r4/Delay  Orientation=down  en=off  latency=1  dbl_ovrd=off  reg_retiming=off  block_type=delay
      settings: infoedit=Hardware notes: A delay line is a chain, each link of which is an SRL16 followed by a flip-flop. If register retiming is enabled, the delay line is a chain of flip-flops.  block_version=8.2
  Delay1 : xbsIndex_r4/Delay  Orientation=down  en=off  latency=1  dbl_ovrd=off  reg_retiming=off  block_type=delay
      settings: infoedit=Hardware notes: A delay line is a chain, each link of which is an SRL16 followed by a flip-flop. If register retiming is enabled, the delay line is a chain of flip-flops.  block_version=8.2
  Delay2 : xbsIndex_r4/Delay  Orientation=down  en=off  latency=1  dbl_ovrd=off  reg_retiming=off  block_type=delay
      settings: infoedit=Hardware notes: A delay line is a chain, each link of which is an SRL16 followed by a flip-flop. If register retiming is enabled, the delay line is a chain of flip-flops.  block_version=8.2
  Display1 : Display
  Display2 : Display
  Display3 : Display
  Down Sample{,1..3} (4 alike) : xbsIndex_r4/Down Sample  sample_ratio=4  sample_phase="Last Value of Frame  (most efficient)"  en=off  latency=1  dbl_ovrd=off  block_type=dsamp
      settings: block_version=8.2
  Gateway Out : xbsIndex_r4/Gateway Out  hdl_port=off  timing_constraint=None  locs_specified=off  LOCs={}  block_type=gatewayout
      settings: infoedit="Gateway out block.  Converts Xilinx fixed point inputs into ouputs of type Simulink integer, double, or fixed point.<P><P>Hardware notes:  In hardware these blocks become top level output ports or are discarded, depending on how they are configured."  block_version=8.2
  Gateway Out1 : xbsIndex_r4/Gateway Out  hdl_port=off  timing_constraint=None  locs_specified=off  LOCs={}  block_type=gatewayout
      settings: infoedit="Gateway out block.  Converts Xilinx fixed point inputs into ouputs of type Simulink integer, double, or fixed point.<P><P>Hardware notes:  In hardware these blocks become top level output ports or are discarded, depending on how they are configured."  block_version=8.2
  I Accumulator : Subsystem
  MAC : Subsystem
  MAC1 : Subsystem
  MAC2 : Subsystem
  MAC3 : Subsystem
  Q Accumulator : Subsystem
  Real-Imag to Complex : RealImagToComplex
  Scope : Scope
  Q Out : Outport
  I Out : Outport  Port=2
  wires:
  Data In/1 -> Down Sample/1, Delay/1, Display1/1
  Delay/1 -> Down Sample1/1, Delay1/1
  Delay1/1 -> Down Sample2/1, Delay2/1
  Delay2/1 -> Down Sample3/1, Display2/1
  Coef0/1 -> MAC/4(Coeff)
  Coef1/1 -> MAC1/4(Coeff)
  I Accumulator/1(Out) -> I Out/1, Gateway Out/1
  Counter/1 -> MAC3/1(Count), MAC2/1(Count), MAC1/1(Count), MAC/1(Count), Q Accumulator/1(Count), I Accumulator/1(Count)
  Coef2/1 -> MAC2/4(Coeff)
  Coef3/1 -> MAC3/4(Coeff)
  Q Accumulator/1(Out) -> Q Out/1, Gateway Out1/1
  Down Sample/1 -> MAC/2(Data In), MAC2/3(Symm Data)
  Down Sample1/1 -> MAC1/3(Symm Data), MAC1/2(Data In)
  Down Sample2/1 -> MAC/3(Symm Data), MAC2/2(Data In)
  Down Sample3/1 -> MAC3/3(Symm Data), MAC3/2(Data In), Display3/1
  MAC/1(Out) -> MAC2/5(PCIN)
  MAC2/1(Out) -> Q Accumulator/2(Sum)
  MAC1/1(Out) -> MAC3/5(PCIN)
  MAC3/1(Out) -> I Accumulator/2(Sum)
  Counter Inv/1 -> MAC/5(Count Inv), MAC1/5(Count Inv), MAC2/6(Counter Inv), MAC3/6(Count Inv)
  Real-Imag to Complex/1 -> Complex to Magnitude-Angle/1
  Complex to Magnitude-Angle/1 -> Scope/1
  Gateway Out/1 -> Real-Imag to Complex/1
  Gateway Out1/1 -> Real-Imag to Complex/2

== system Casc_Filter_x4/DDC/DDC A1/Gaussian FIR Filters ==
  Counter : Inport
  Counter Inv : Inport  Port=2
  Q In : Inport  Port=3
  Coef0 : Inport  Port=4
  Coef1 : Inport  Port=5
  Coef2 : Inport  Port=6
  I In : Inport  Port=7
  Gaussian FIR Filter : Subsystem
  Gaussian FIR Filter1 : Subsystem
  I Out : Outport
  Q Out : Outport  Port=2
  wires:
  Counter/1 -> Gaussian FIR Filter/1(Counter), Gaussian FIR Filter1/1(Counter)
  Counter Inv/1 -> Gaussian FIR Filter/2(Counter Inv), Gaussian FIR Filter1/2(Counter Inv)
  Q In/1 -> Gaussian FIR Filter/3(Data In)
  I In/1 -> Gaussian FIR Filter1/3(Data In)
  Gaussian FIR Filter/1(Data Out) -> Q Out/1
  Gaussian FIR Filter1/1(Data Out) -> I Out/1
  Coef0/1 -> Gaussian FIR Filter/4(Coef0), Gaussian FIR Filter1/4(Coef0)
  Coef1/1 -> Gaussian FIR Filter/5(Coef1), Gaussian FIR Filter1/5(Coef1)
  Coef2/1 -> Gaussian FIR Filter/6(Coef2), Gaussian FIR Filter1/6(Coef2)
